simulink model "motorTF"  (R2025b)
settings: Solver=VariableStepAuto  StartTime=0.0  StopTime=10.0  RelTol=1e-3
libraries: metux_library x1
settings Model: DataDictionary=motorData.sldd  Creator=karadeli  LastModifiedBy=karadeli

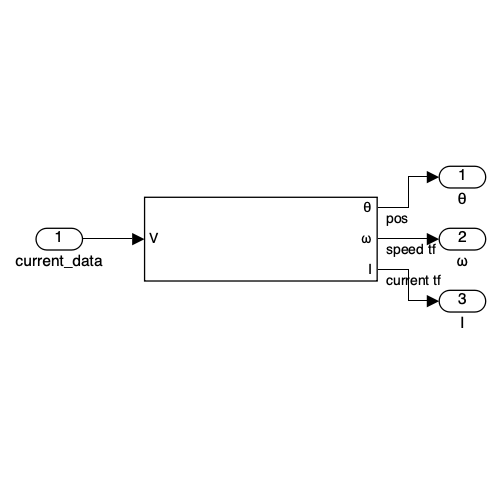
[thumbnail: Simulink's stored preview of the top-level diagram]
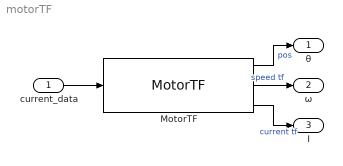
== system motorTF ==
  current_data : Inport  Unit=V
  MotorTF : metux_library/MotorTF  SystemSampleTime=-1  VariantActivationTime=update diagram  EmptyChoice=off  PassThrough=off  PassThroughVariantControl=(default)  EmptyChoiceVariantControl=(default)  AllowFlexibleInterface=on  Latency=0  AutoFrameSizeCalculation=off
  θ : Outport  Unit=deg
  ω : Outport  Port=2  Unit=deg/s
  I : Outport  Port=3  Unit=A
  wires:
  current_data/1 -> MotorTF/1
  MotorTF/1 -> θ/1  "pos"
  MotorTF/2 -> ω/1  "speed tf"
  MotorTF/3 -> I/1  "current tf"
